simulink model "Simulink1"  (R2014a)
settings: Solver=ode45  StartTime=0.0  StopTime=10.0  RelTol=1e-3
settings Model: Creator=MS  LastModifiedBy=MS

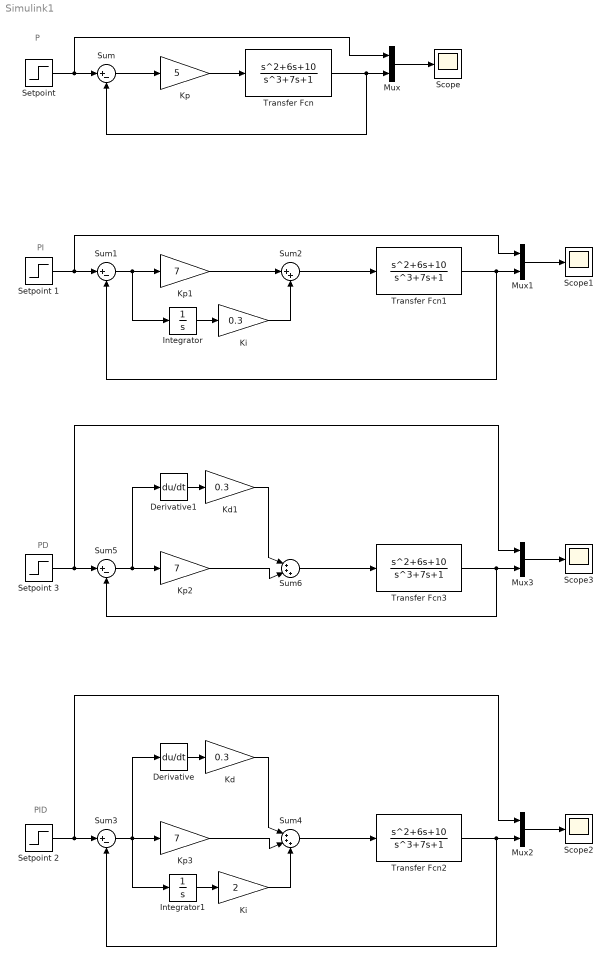
== system Simulink1 ==
  note: PI
  note: PD
  note: PID
  note: P
  Derivative : Derivative
  Derivative1 : Derivative
  Integrator : Integrator
  Integrator1 : Integrator
  Kd : Gain  Gain=0.3
  Kd1 : Gain  Gain=0.3
  Ki : Gain  Gain=2
  "Ki " : Gain  Gain=0.3
  Kp : Gain  Gain=5
  Kp1 : Gain  Gain=7
  Kp2 : Gain  Gain=7
  Kp3 : Gain  Gain=7
  Mux{,1..3} (4 alike) : Mux  Inputs=2
  Scope{,1..3} (4 alike) : Scope
      Scope settings: YMax=350
      Scope1 settings: YMax=350
      Scope2 settings: YMax=350  SaveName=ScopeData2
      Scope3 settings: YMax=350  SaveName=ScopeData3
  Setpoint {,1..3} (4 alike) : Step  Time=0  After=0.3  SampleTime=0
  Sum{,1,3,5} (4 alike) : Sum  Inputs=|+-
  Sum2 : Sum  Inputs=|++
  Sum4 : Sum  Inputs=|+++
  Sum6 : Sum  Inputs=|+++
  Transfer Fcn{,1..3} (4 alike) : TransferFcn  Numerator=[1,6,10]  Denominator=[1,0,7,1]
  wires:
  Transfer Fcn/1 -> Mux/2, Sum/2
  Kp/1 -> Transfer Fcn/1
  Sum/1 -> Kp/1
  "Setpoint "/1 -> Mux/1, Sum/1
  Mux/1 -> Scope/1
  Transfer Fcn1/1 -> Mux1/2, Sum1/2
  Sum1/1 -> Integrator/1, Kp1/1
  Setpoint 1/1 -> Mux1/1, Sum1/1
  Mux1/1 -> Scope1/1
  Integrator/1 -> "Ki "/1
  Kp1/1 -> Sum2/1
  Sum2/1 -> Transfer Fcn1/1
  "Ki "/1 -> Sum2/2
  Transfer Fcn2/1 -> Mux2/2, Sum3/2
  Sum3/1 -> Derivative/1, Integrator1/1, Kp3/1
  Setpoint 2/1 -> Mux2/1, Sum3/1
  Mux2/1 -> Scope2/1
  Integrator1/1 -> Ki/1
  Kp3/1 -> Sum4/2
  Sum4/1 -> Transfer Fcn2/1
  Ki/1 -> Sum4/3
  Derivative/1 -> Kd/1
  Kd/1 -> Sum4/1
  Transfer Fcn3/1 -> Mux3/2, Sum5/2
  Sum5/1 -> Derivative1/1, Kp2/1
  Setpoint 3/1 -> Mux3/1, Sum5/1
  Mux3/1 -> Scope3/1
  Kp2/1 -> Sum6/2
  Sum6/1 -> Transfer Fcn3/1
  Derivative1/1 -> Kd1/1
  Kd1/1 -> Sum6/1
